simulink model "SimulationV4"  (R2018a)
settings: Solver=ode45  StartTime=0.0  StopTime=tfin  FixedStep=0.001  RelTol=1e-09  EnableMultiTasking=on
values from neighbouring files (symbols this model uses):
  A = eval(subs(A))    [CalculTFs.m]    (also in EquationCapteur.m = length(a); Modelisation.m = subs(A, [thetaeq, phieq], [0, 0]); modelisation.m = [[zeros([3,3]) eye(3) zeros([3,2]) zeros([3,2]) zeros([3,3]); run_bancessai.m)
  A_phi = [A_plaque(1,1) A_plaque(1,4) A_plaque(1,7) ... (first row only)    [CalculTFs.m]
  A_theta = [A_plaque(2,2) A_plaque(2,5) A_plaque(2,8) ... (first row only)    [CalculTFs.m]
  A_z = [A_plaque(3,3) A_plaque(3,6) A_plaque(3,9) ... (first row only)    [CalculTFs.m]
  ae0 = a2(1)    [Actionneurs.m]    (also in CoefficientsActionneurs.mat = 1.33340598826)
  ae1 = a2(2)    [Actionneurs.m]    (also in CoefficientsActionneurs.mat = 362.21410211)
  ae2 = a2(3)    [Actionneurs.m]    (also in CoefficientsActionneurs.mat = 2183.40136704)
  ae3 = a2(4)    [Actionneurs.m]    (also in CoefficientsActionneurs.mat = 705425.288236)
  as0 = a3(1)    [Actionneurs.m]    (also in CoefficientsActionneurs.mat = 0.0586667067)
  as1 = a3(2)    [Actionneurs.m]    (also in CoefficientsActionneurs.mat = 22.4105523392)
  as2 = a3(3)    [Actionneurs.m]    (also in CoefficientsActionneurs.mat = 860.394175869)
  as3 = a3(4)    [Actionneurs.m]    (also in CoefficientsActionneurs.mat = 233710.908706)
  B = eval(subs(B))    [CalculTFs.m]    (also in EquationCapteur.m = length(b); Modelisation.m = [[zeros([3,3])]; modelisation.m = [[zeros([3,3])]; run_bancessai.m)
  B_phi = [0;0;B_plaque(7,1)]    [CalculTFs.m]
  B_theta = [0;0;B_plaque(8,2)]    [CalculTFs.m]
  B_z = [0;0;B_plaque(9,3)]    [CalculTFs.m]
  be1 = 13.029359254409743    (= 13.0293592544)    [Actionneurs.m]    (also in CoefficientsActionneurs.mat)
  C = eval(subs(C))    [CalculTFs.m]    (also in EquationCapteur.m = length(c); Modelisation.m = [[Tdef zeros([3,3]) zeros([3,4]) zeros([3,3])]; modelisation.m = [[Tdef zeros([3,3]) zeros([3,4]) zeros([3,3])]; run_bancessai.m)
  C_dec = [1 0 0]    [CalculTFs.m]
  D = eval(subs(D))    [CalculTFs.m]    (also in EquationCapteur.m = length(d); Linearisation.mat = [0 0 0 0 0 0 0 0 0 0 0 0 ... (21 elements, 7x3)]; Modelisation.m = zeros([7,3]); modelisation.m = zeros([7,3]))
  D_dec = [0]    [CalculTFs.m]
  g = 9.81    [bancEssaiConstantes.m]    (also in trajectoire.m = sqrt(1 + (df).^2))
  Jx = 1169e-06    (= 0.001169)    [bancEssaiConstantes.m]
  Jy = Jx    (= 0.001169)    [bancEssaiConstantes.m]
  LA = LL    (= 0.115)    [bancEssaiConstantes.m]
  LB = LL    (= 0.115)    [bancEssaiConstantes.m]
  LC = LL    (= 0.115)    [bancEssaiConstantes.m]
  mS = 0.0080    (= 0.008)    [bancEssaiConstantes.m]
  mSeff = mS+JS/rS^2    (= 0.0112)    [bancEssaiConstantes.m]
  mtot = mP + sig*mS    [bancEssaiConstantes.m]
  Pxeq = xSeq    [equilibre.m]    (also in equilibre_cube.m)
  Pyeq = ySeq    [equilibre.m]    (also in equilibre_cube.m)
  Pzeq = .015    (= 0.015)    [run_bancessai.m]
  RA = RR    (= 3.6)    [bancEssaiConstantes.m]
  RB = RR    (= 3.6)    [bancEssaiConstantes.m]
  RC = RR    (= 3.6)    [bancEssaiConstantes.m]
  sig = 1    [run_bancessai.m]
  TDEF = [yvec_DEF'; -xvec_DEF'; ones(1,3)]    [bancEssaiConstantes.m]
  U = [YA YB YC ... (first row only)    [bancEssaiConstantes.m]
  VAeq = double(IAeq*RA)    [equilibre.m]    (also in equilibre_cube.m = double(IAeq/RA))
  VBeq = double(IBeq*RB)    [equilibre.m]    (also in equilibre_cube.m = double(IBeq/RB))
  VCeq = double(ICeq*RC)    [equilibre.m]    (also in equilibre_cube.m = double(ICeq/RC))
  Vmax = 16.0    (= 16)    [bancEssaiConstantes.m]
  XA = +rABC    (= 0.0952)    [bancEssaiConstantes.m]
  XB = -rABC*sind(30)    [bancEssaiConstantes.m]
  XC = -rABC*sind(30)    [bancEssaiConstantes.m]
  XD = +rDEF*sind(30)    [bancEssaiConstantes.m]
  XE = -rDEF    (= -0.08)    [bancEssaiConstantes.m]
  XF = +rDEF*sind(30)    [bancEssaiConstantes.m]
  YA = 0.0    (= 0)    [bancEssaiConstantes.m]
  YB = +rABC*cosd(30)    [bancEssaiConstantes.m]
  YC = -rABC*cosd(30)    [bancEssaiConstantes.m]
  YD = +rDEF*cosd(30)    [bancEssaiConstantes.m]
  YE = 0.0    (= 0)    [bancEssaiConstantes.m]
  YF = -rDEF*cosd(30)    [bancEssaiConstantes.m]
undefined symbols (not defined in the file or in its folder): A_sphere, B_sphere, C_sphere, D_sphere
(part 2 of 2)

== system SimulationV4/Asservissements2/__InputSSForSFun__ ==
  zD : Inport
  zE : Inport  Port=2
  zF : Inport  Port=3
  Axdes : Inport  Port=4
  Aydes : Inport  Port=5
  zdes : Inport  Port=6
  xdes : Inport  Port=7
  ydes : Inport  Port=8
  Px : Inport  Port=9
  Py : Inport  Port=10
  Vx : Inport  Port=11
  Vy : Inport  Port=12
  __UniqueOutportName__1__ : Outport
  __UniqueOutportName__2__ : Outport  Port=2
  __UniqueOutportName__3__ : Outport  Port=3
  __UniqueOutportName__4__ : Outport  Port=4
  __UniqueOutportName__5__ : Outport  Port=5
  __UniqueOutportName__6__ : Outport  Port=6
  __UniqueOutportName__7__ : Outport  Port=7
  __UniqueOutportName__8__ : Outport  Port=8
  __UniqueOutportName__9__ : Outport  Port=9
  __UniqueOutportName__10__ : Outport  Port=10
  __UniqueOutportName__11__ : Outport  Port=11
  __UniqueOutportName__12__ : Outport  Port=12
  wires:
  zD/1 -> __UniqueOutportName__1__/1
  zE/1 -> __UniqueOutportName__2__/1
  zF/1 -> __UniqueOutportName__3__/1
  Axdes/1 -> __UniqueOutportName__4__/1
  Aydes/1 -> __UniqueOutportName__5__/1
  zdes/1 -> __UniqueOutportName__6__/1
  xdes/1 -> __UniqueOutportName__7__/1
  ydes/1 -> __UniqueOutportName__8__/1
  Px/1 -> __UniqueOutportName__9__/1
  Py/1 -> __UniqueOutportName__10__/1
  Vx/1 -> __UniqueOutportName__11__/1
  Vy/1 -> __UniqueOutportName__12__/1

== system SimulationV4/Asservissements2/__OutputSSForSFun__ ==
  __UniqueInportName__1__ : Inport
  __UniqueInportName__2__ : Inport  Port=2
  __UniqueInportName__3__ : Inport  Port=3
  __UniqueInportName__4__ : Inport  Port=4
  __UniqueInportName__5__ : Inport  Port=5
  VAcalcule : Outport
  VBcalcule : Outport  Port=2
  VCcalcule : Outport  Port=3
  Axcalcule : Outport  Port=4
  Aycalcule : Outport  Port=5
  wires:
  __UniqueInportName__1__/1 -> VAcalcule/1
  __UniqueInportName__2__/1 -> VBcalcule/1
  __UniqueInportName__3__/1 -> VCcalcule/1
  __UniqueInportName__4__/1 -> Axcalcule/1  "Ax_des"
  __UniqueInportName__5__/1 -> Aycalcule/1  "Ay_des"

== system SimulationV4/Asservissements3/__InputSSForSFun__ ==
  zD : Inport
  zE : Inport  Port=2
  zF : Inport  Port=3
  Axdes : Inport  Port=4
  Aydes : Inport  Port=5
  zdes : Inport  Port=6
  xdes : Inport  Port=7
  ydes : Inport  Port=8
  Px : Inport  Port=9
  Py : Inport  Port=10
  Vx : Inport  Port=11
  Vy : Inport  Port=12
  __UniqueOutportName__1__ : Outport
  __UniqueOutportName__2__ : Outport  Port=2
  __UniqueOutportName__3__ : Outport  Port=3
  __UniqueOutportName__4__ : Outport  Port=4
  __UniqueOutportName__5__ : Outport  Port=5
  __UniqueOutportName__6__ : Outport  Port=6
  __UniqueOutportName__7__ : Outport  Port=7
  __UniqueOutportName__8__ : Outport  Port=8
  __UniqueOutportName__9__ : Outport  Port=9
  __UniqueOutportName__10__ : Outport  Port=10
  __UniqueOutportName__11__ : Outport  Port=11
  __UniqueOutportName__12__ : Outport  Port=12
  wires:
  zD/1 -> __UniqueOutportName__1__/1
  zE/1 -> __UniqueOutportName__2__/1
  zF/1 -> __UniqueOutportName__3__/1
  Axdes/1 -> __UniqueOutportName__4__/1
  Aydes/1 -> __UniqueOutportName__5__/1
  zdes/1 -> __UniqueOutportName__6__/1
  xdes/1 -> __UniqueOutportName__7__/1
  ydes/1 -> __UniqueOutportName__8__/1
  Px/1 -> __UniqueOutportName__9__/1
  Py/1 -> __UniqueOutportName__10__/1
  Vx/1 -> __UniqueOutportName__11__/1
  Vy/1 -> __UniqueOutportName__12__/1

== system SimulationV4/Asservissements3/__OutputSSForSFun__ ==
  __UniqueInportName__1__ : Inport
  __UniqueInportName__2__ : Inport  Port=2
  __UniqueInportName__3__ : Inport  Port=3
  __UniqueInportName__4__ : Inport  Port=4
  __UniqueInportName__5__ : Inport  Port=5
  VAcalcule : Outport
  VBcalcule : Outport  Port=2
  VCcalcule : Outport  Port=3
  Axcalcule : Outport  Port=4
  Aycalcule : Outport  Port=5
  wires:
  __UniqueInportName__1__/1 -> VAcalcule/1
  __UniqueInportName__2__/1 -> VBcalcule/1
  __UniqueInportName__3__/1 -> VCcalcule/1
  __UniqueInportName__4__/1 -> Axcalcule/1  "Ax_des"
  __UniqueInportName__5__/1 -> Aycalcule/1  "Ay_des"

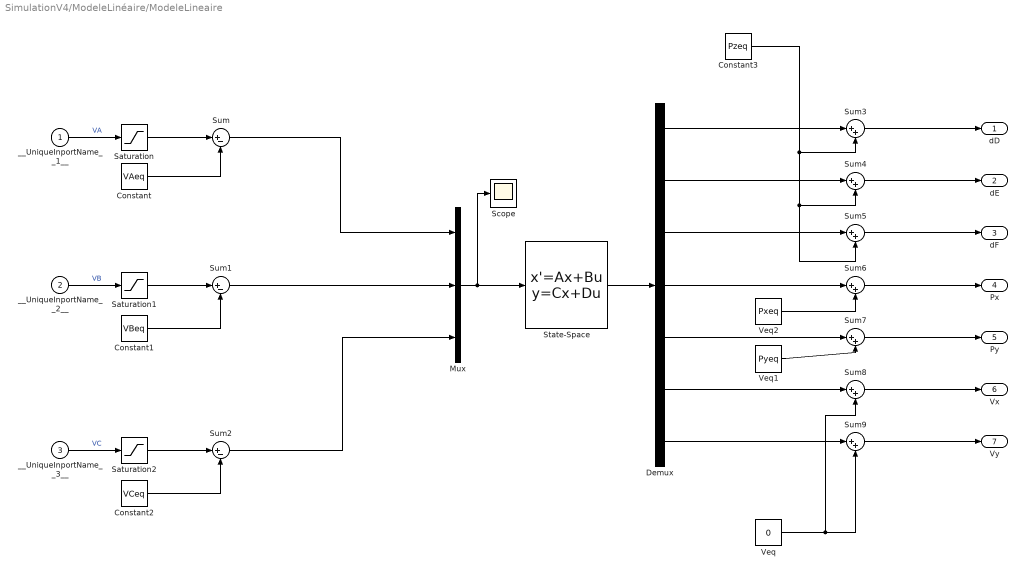
== system SimulationV4/ModeleLinéaire/ModeleLineaire ==
  __UniqueInportName__1__ : Inport
  __UniqueInportName__2__ : Inport  Port=2
  __UniqueInportName__3__ : Inport  Port=3
  Constant : Constant  Value=VAeq
  Constant1 : Constant  Value=VBeq
  Constant2 : Constant  Value=VCeq
  Constant3 : Constant  Value=Pzeq
  Demux : Demux  Outputs=7
  Mux : Mux  Inputs=3
  Saturation : Saturate  UpperLimit=Vmax  LowerLimit=-Vmax
  Saturation1 : Saturate  UpperLimit=Vmax  LowerLimit=-Vmax
  Saturation2 : Saturate  UpperLimit=Vmax  LowerLimit=-Vmax
  Scope : Scope
  State-Space : StateSpace  A=A  B=B  C=C  D=D  InitialCondition=0
  Sum : Sum  Inputs=|+-
  Sum1 : Sum  Inputs=|+-
  Sum2 : Sum  Inputs=|+-
  Sum{3..9} (7 alike) : Sum  Inputs=|++
  Veq : Constant  Value=0
  Veq1 : Constant  Value=Pyeq
  Veq2 : Constant  Value=Pxeq
  dD : Outport
  dE : Outport  Port=2
  dF : Outport  Port=3
  Px : Outport  Port=4
  Py : Outport  Port=5
  Vx : Outport  Port=6
  Vy : Outport  Port=7
  wires:
  __UniqueInportName__1__/1 -> Saturation/1  "VA"
  __UniqueInportName__2__/1 -> Saturation1/1  "VB"
  __UniqueInportName__3__/1 -> Saturation2/1  "VC"
  Mux/1 -> State-Space/1, Scope/1
  State-Space/1 -> Demux/1
  Constant/1 -> Sum/2
  Saturation/1 -> Sum/1
  Sum/1 -> Mux/1
  Saturation1/1 -> Sum1/1
  Constant1/1 -> Sum1/2
  Sum1/1 -> Mux/2
  Constant2/1 -> Sum2/2
  Sum2/1 -> Mux/3
  Saturation2/1 -> Sum2/1
  Sum3/1 -> dD/1
  Sum4/1 -> dE/1
  Sum5/1 -> dF/1
  Sum6/1 -> Px/1
  Sum7/1 -> Py/1
  Sum8/1 -> Vx/1
  Sum9/1 -> Vy/1
  Veq/1 -> Sum8/2, Sum9/2
  Demux/7 -> Sum9/1
  Demux/6 -> Sum8/1
  Veq1/1 -> Sum7/2
  Demux/5 -> Sum7/1
  Veq2/1 -> Sum6/2
  Demux/4 -> Sum6/1
  Constant3/1 -> Sum3/2, Sum4/2, Sum5/2
  Demux/1 -> Sum3/1
  Demux/2 -> Sum4/1
  Demux/3 -> Sum5/1

== system SimulationV4/ModeleLinéaire/__InputSSForSFun__ ==
  VAdesire : Inport
  VBdesire : Inport  Port=2
  VCdesire : Inport  Port=3
  __UniqueOutportName__1__ : Outport
  __UniqueOutportName__2__ : Outport  Port=2
  __UniqueOutportName__3__ : Outport  Port=3
  wires:
  VAdesire/1 -> __UniqueOutportName__1__/1
  VBdesire/1 -> __UniqueOutportName__2__/1
  VCdesire/1 -> __UniqueOutportName__3__/1

== system SimulationV4/ModeleLinéaire/__OutputSSForSFun__ ==
  __UniqueInportName__17__ : Inport
  __UniqueInportName__18__ : Inport  Port=2
  __UniqueInportName__19__ : Inport  Port=3
  __UniqueInportName__7__ : Inport  Port=4
  __UniqueInportName__8__ : Inport  Port=5
  __UniqueInportName__9__ : Inport  Port=6
  __UniqueInportName__10__ : Inport  Port=7
  zD : Outport
  zE : Outport  Port=2
  zF : Outport  Port=3
  Px : Outport  Port=4
  Py : Outport  Port=5
  Vx : Outport  Port=6
  Vy : Outport  Port=7
  wires:
  __UniqueInportName__7__/1 -> Px/1  "Px"
  __UniqueInportName__8__/1 -> Py/1  "Py"
  __UniqueInportName__9__/1 -> Vx/1  "Vx"
  __UniqueInportName__10__/1 -> Vy/1  "Vy"
  __UniqueInportName__17__/1 -> zD/1  "zd"
  __UniqueInportName__18__/1 -> zE/1  "ze"
  __UniqueInportName__19__/1 -> zF/1  "zf"

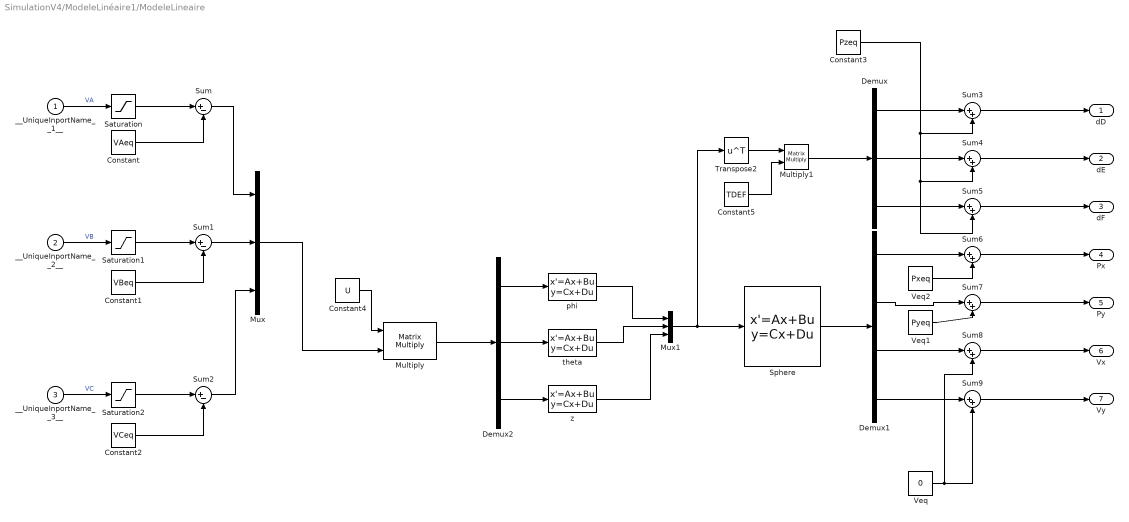
== system SimulationV4/ModeleLinéaire1/ModeleLineaire ==
  __UniqueInportName__1__ : Inport
  __UniqueInportName__2__ : Inport  Port=2
  __UniqueInportName__3__ : Inport  Port=3
  Constant : Constant  Value=VAeq
  Constant1 : Constant  Value=VBeq
  Constant2 : Constant  Value=VCeq
  Constant3 : Constant  Value=Pzeq
  Constant4 : Constant  Value=U
  Constant5 : Constant  Value=TDEF
  Demux : Demux  Outputs=3
  Demux1 : Demux
  Demux2 : Demux  Outputs=3
  Multiply : Product  Multiplication=Matrix(*)  OutDataTypeStr=Inherit: Same as first input
  Multiply1 : Product  Multiplication=Matrix(*)
  Mux : Mux  Inputs=3
  Mux1 : Mux  Inputs=3
  Saturation : Saturate  UpperLimit=Vmax  LowerLimit=-Vmax
  Saturation1 : Saturate  UpperLimit=Vmax  LowerLimit=-Vmax
  Saturation2 : Saturate  UpperLimit=Vmax  LowerLimit=-Vmax
  Sphere : StateSpace  A=A_sphere  B=B_sphere  C=C_sphere  D=D_sphere  InitialCondition=0
  Sum : Sum  Inputs=|+-
  Sum1 : Sum  Inputs=|+-
  Sum2 : Sum  Inputs=|+-
  Sum{3..9} (7 alike) : Sum  Inputs=|++
  Transpose2 : Math  Operator=transpose  SaturateOnIntegerOverflow=on
  Veq : Constant  Value=0
  Veq1 : Constant  Value=Pyeq
  Veq2 : Constant  Value=Pxeq
  phi : StateSpace  A=A_phi  B=B_phi  C=C_dec  D=D_dec  InitialCondition=0
  theta : StateSpace  A=A_theta  B=B_theta  C=C_dec  D=D_dec  InitialCondition=0
  z : StateSpace  A=A_z  B=B_z  C=C_dec  D=D_dec  InitialCondition=0
  dD : Outport
  dE : Outport  Port=2
  dF : Outport  Port=3
  Px : Outport  Port=4
  Py : Outport  Port=5
  Vx : Outport  Port=6
  Vy : Outport  Port=7
  wires:
  __UniqueInportName__1__/1 -> Saturation/1  "VA"
  __UniqueInportName__2__/1 -> Saturation1/1  "VB"
  __UniqueInportName__3__/1 -> Saturation2/1  "VC"
  Sphere/1 -> Demux1/1
  Constant/1 -> Sum/2
  Saturation/1 -> Sum/1
  Sum/1 -> Mux/1
  Saturation1/1 -> Sum1/1
  Constant1/1 -> Sum1/2
  Sum1/1 -> Mux/2
  Constant2/1 -> Sum2/2
  Sum2/1 -> Mux/3
  Saturation2/1 -> Sum2/1
  Sum3/1 -> dD/1
  Sum4/1 -> dE/1
  Sum5/1 -> dF/1
  Sum6/1 -> Px/1
  Sum7/1 -> Py/1
  Sum8/1 -> Vx/1
  Sum9/1 -> Vy/1
  Veq/1 -> Sum8/2, Sum9/2
  Demux1/4 -> Sum9/1
  Demux1/3 -> Sum8/1
  Veq1/1 -> Sum7/2
  Demux1/2 -> Sum7/1
  Veq2/1 -> Sum6/2
  Demux1/1 -> Sum6/1
  Constant3/1 -> Sum3/2, Sum4/2, Sum5/2
  Demux/1 -> Sum3/1
  Demux/2 -> Sum4/1
  Demux/3 -> Sum5/1
  Mux/1 -> Multiply/2
  Constant4/1 -> Multiply/1
  Multiply/1 -> Demux2/1
  Multiply1/1 -> Demux/1
  Constant5/1 -> Multiply1/2
  Transpose2/1 -> Multiply1/1
  Mux1/1 -> Transpose2/1, Sphere/1
  phi/1 -> Mux1/1
  theta/1 -> Mux1/2
  z/1 -> Mux1/3
  Demux2/1 -> phi/1
  Demux2/2 -> theta/1
  Demux2/3 -> z/1

== system SimulationV4/ModeleLinéaire1/__InputSSForSFun__ ==
  VAdesire : Inport
  VBdesire : Inport  Port=2
  VCdesire : Inport  Port=3
  __UniqueOutportName__1__ : Outport
  __UniqueOutportName__2__ : Outport  Port=2
  __UniqueOutportName__3__ : Outport  Port=3
  wires:
  VAdesire/1 -> __UniqueOutportName__1__/1
  VBdesire/1 -> __UniqueOutportName__2__/1
  VCdesire/1 -> __UniqueOutportName__3__/1

== system SimulationV4/ModeleLinéaire1/__OutputSSForSFun__ ==
  __UniqueInportName__17__ : Inport
  __UniqueInportName__18__ : Inport  Port=2
  __UniqueInportName__19__ : Inport  Port=3
  __UniqueInportName__7__ : Inport  Port=4
  __UniqueInportName__8__ : Inport  Port=5
  __UniqueInportName__9__ : Inport  Port=6
  __UniqueInportName__10__ : Inport  Port=7
  zD : Outport
  zE : Outport  Port=2
  zF : Outport  Port=3
  Px : Outport  Port=4
  Py : Outport  Port=5
  Vx : Outport  Port=6
  Vy : Outport  Port=7
  wires:
  __UniqueInportName__7__/1 -> Px/1  "Px"
  __UniqueInportName__8__/1 -> Py/1  "Py"
  __UniqueInportName__9__/1 -> Vx/1  "Vx"
  __UniqueInportName__10__/1 -> Vy/1  "Vy"
  __UniqueInportName__17__/1 -> zD/1  "zd"
  __UniqueInportName__18__/1 -> zE/1  "ze"
  __UniqueInportName__19__/1 -> zF/1  "zf"

== system SimulationV4/ModeleNonLineaire/__InputSSForSFun__ ==
  VAdesire : Inport
  VBdesire : Inport  Port=2
  VCdesire : Inport  Port=3
  __UniqueOutportName__1__ : Outport
  __UniqueOutportName__2__ : Outport  Port=2
  __UniqueOutportName__3__ : Outport  Port=3
  wires:
  VAdesire/1 -> __UniqueOutportName__1__/1
  VBdesire/1 -> __UniqueOutportName__2__/1
  VCdesire/1 -> __UniqueOutportName__3__/1

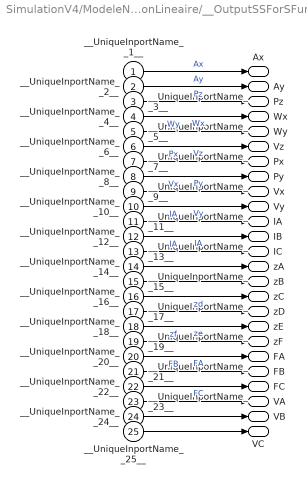
== system SimulationV4/ModeleNonLineaire/__OutputSSForSFun__ ==
  __UniqueInportName__1__ : Inport
  __UniqueInportName__2__ : Inport  Port=2
  __UniqueInportName__3__ : Inport  Port=3
  __UniqueInportName__4__ : Inport  Port=4
  __UniqueInportName__5__ : Inport  Port=5
  __UniqueInportName__6__ : Inport  Port=6
  __UniqueInportName__7__ : Inport  Port=7
  __UniqueInportName__8__ : Inport  Port=8
  __UniqueInportName__9__ : Inport  Port=9
  __UniqueInportName__10__ : Inport  Port=10
  __UniqueInportName__11__ : Inport  Port=11
  __UniqueInportName__12__ : Inport  Port=12
  __UniqueInportName__13__ : Inport  Port=13
  __UniqueInportName__14__ : Inport  Port=14
  __UniqueInportName__15__ : Inport  Port=15
  __UniqueInportName__16__ : Inport  Port=16
  __UniqueInportName__17__ : Inport  Port=17
  __UniqueInportName__18__ : Inport  Port=18
  __UniqueInportName__19__ : Inport  Port=19
  __UniqueInportName__20__ : Inport  Port=20
  __UniqueInportName__21__ : Inport  Port=21
  __UniqueInportName__22__ : Inport  Port=22
  __UniqueInportName__23__ : Inport  Port=23
  __UniqueInportName__24__ : Inport  Port=24
  __UniqueInportName__25__ : Inport  Port=25
  Ax : Outport
  Ay : Outport  Port=2
  Pz : Outport  Port=3
  Wx : Outport  Port=4
  Wy : Outport  Port=5
  Vz : Outport  Port=6
  Px : Outport  Port=7
  Py : Outport  Port=8
  Vx : Outport  Port=9
  Vy : Outport  Port=10
  IA : Outport  Port=11
  IB : Outport  Port=12
  IC : Outport  Port=13
  zA : Outport  Port=14
  zB : Outport  Port=15
  zC : Outport  Port=16
  zD : Outport  Port=17
  zE : Outport  Port=18
  zF : Outport  Port=19
  FA : Outport  Port=20
  FB : Outport  Port=21
  FC : Outport  Port=22
  VA : Outport  Port=23
  VB : Outport  Port=24
  VC : Outport  Port=25
  wires:
  __UniqueInportName__1__/1 -> Ax/1  "Ax"
  __UniqueInportName__2__/1 -> Ay/1  "Ay"
  __UniqueInportName__3__/1 -> Pz/1  "Pz"
  __UniqueInportName__4__/1 -> Wx/1  "Wx"
  __UniqueInportName__5__/1 -> Wy/1  "Wy"
  __UniqueInportName__6__/1 -> Vz/1  "Vz"
  __UniqueInportName__7__/1 -> Px/1  "Px"
  __UniqueInportName__8__/1 -> Py/1  "Py"
  __UniqueInportName__9__/1 -> Vx/1  "Vx"
  __UniqueInportName__10__/1 -> Vy/1  "Vy"
  __UniqueInportName__11__/1 -> IA/1  "IA"
  __UniqueInportName__12__/1 -> IB/1  "IA"
  __UniqueInportName__13__/1 -> IC/1  "IA"
  __UniqueInportName__14__/1 -> zA/1
  __UniqueInportName__15__/1 -> zB/1
  __UniqueInportName__16__/1 -> zC/1
  __UniqueInportName__17__/1 -> zD/1  "zd"
  __UniqueInportName__18__/1 -> zE/1  "ze"
  __UniqueInportName__19__/1 -> zF/1  "zf"
  __UniqueInportName__20__/1 -> FA/1  "FA"
  __UniqueInportName__21__/1 -> FB/1  "FB"
  __UniqueInportName__22__/1 -> FC/1  "FC"
  __UniqueInportName__23__/1 -> VA/1
  __UniqueInportName__24__/1 -> VB/1
  __UniqueInportName__25__/1 -> VC/1

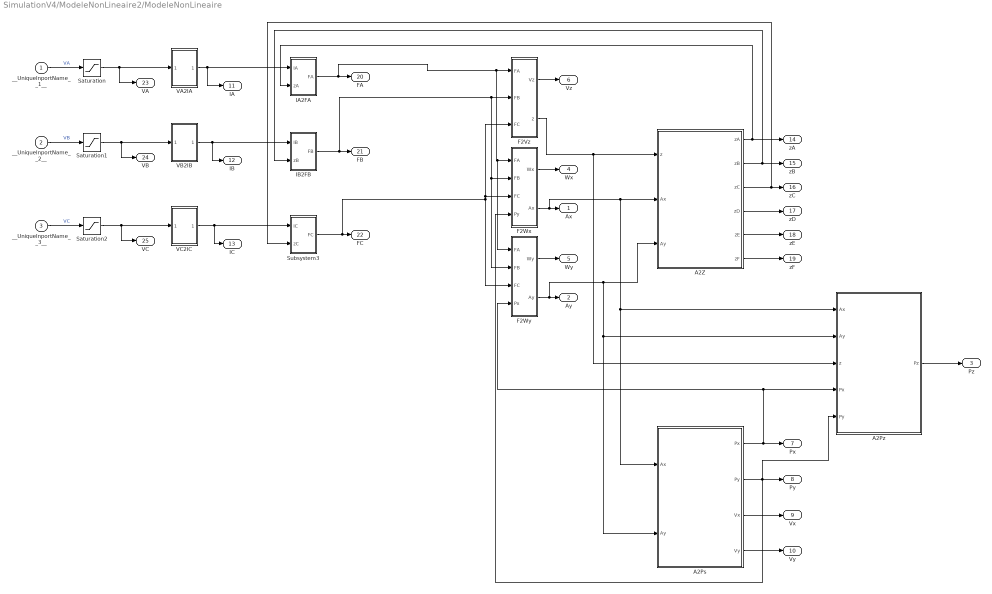
== system SimulationV4/ModeleNonLineaire2/ModeleNonLineaire ==
  __UniqueInportName__1__ : Inport
  __UniqueInportName__2__ : Inport  Port=2
  __UniqueInportName__3__ : Inport  Port=3
  A2Ps : Subsystem
  A2Pz : Subsystem
  A2Z : Subsystem
  F2Vz : Subsystem
  F2Wx : Subsystem
  F2Wy : Subsystem
  IA2FA : Subsystem
  IB2FB : Subsystem
  Saturation : Saturate  UpperLimit=Vmax  LowerLimit=-Vmax
  Saturation1 : Saturate  UpperLimit=Vmax  LowerLimit=-Vmax
  Saturation2 : Saturate  UpperLimit=Vmax  LowerLimit=-Vmax
  Subsystem3 : Subsystem
  VA2IA : Subsystem
  VB2IB : Subsystem
  VC2IC : Subsystem
  Ax : Outport
  Ay : Outport  Port=2
  Pz : Outport  Port=3
  Wx : Outport  Port=4
  Wy : Outport  Port=5
  Vz : Outport  Port=6
  Px : Outport  Port=7
  Py : Outport  Port=8
  Vx : Outport  Port=9
  Vy : Outport  Port=10
  IA : Outport  Port=11
  IB : Outport  Port=12
  IC : Outport  Port=13
  zA : Outport  Port=14
  zB : Outport  Port=15
  zC : Outport  Port=16
  zD : Outport  Port=17
  zE : Outport  Port=18
  zF : Outport  Port=19
  FA : Outport  Port=20
  FB : Outport  Port=21
  FC : Outport  Port=22
  VA : Outport  Port=23
  VB : Outport  Port=24
  VC : Outport  Port=25
  wires:
  __UniqueInportName__1__/1 -> Saturation/1  "VA"
  __UniqueInportName__2__/1 -> Saturation1/1  "VB"
  __UniqueInportName__3__/1 -> Saturation2/1  "VC"
  Saturation/1 -> VA2IA/1(In1), VA/1
  VA2IA/1(Out1) -> IA2FA/1(IA), IA/1
  Saturation1/1 -> VB2IB/1(In1), VB/1
  VB2IB/1(Out1) -> IB/1, IB2FB/1(IB)
  Saturation2/1 -> VC2IC/1(In1), VC/1
  VC2IC/1(Out1) -> Subsystem3/1(IC), IC/1
  F2Vz/1(Vz) -> Vz/1
  F2Wx/1(Wx) -> Wx/1
  F2Wy/1(Wy) -> Wy/1
  IA2FA/1(FA) -> F2Wy/1(FA), F2Wx/1(FA), F2Vz/1(FA), FA/1
  Subsystem3/1(FC) -> F2Vz/3(FC), F2Wx/3(FC), F2Wy/3(FC), FC/1
  IB2FB/1(FB) -> F2Wy/2(FB), F2Wx/2(FB), F2Vz/2(FB), FB/1
  F2Wy/2(Ay) -> A2Ps/2(Ay), A2Pz/2(Ay), A2Z/3(Ay), Ay/1
  F2Vz/2(z) -> A2Pz/3(z), A2Z/1(z)
  F2Wx/2(Ax) -> A2Pz/1(Ax), A2Ps/1(Ax), A2Z/2(Ax), Ax/1
  A2Z/1(zA) -> zA/1, IA2FA/2(zA)
  A2Z/2(zB) -> IB2FB/2(zB), zB/1
  A2Z/3(zC) -> Subsystem3/2(zC), zC/1
  A2Z/4(zD) -> zD/1
  A2Z/5(zE) -> zE/1
  A2Z/6(zF) -> zF/1
  A2Ps/2(Py) -> A2Pz/5(Py), F2Wx/4(Py), Py/1
  A2Ps/3(Vx) -> Vx/1
  A2Ps/4(Vy) -> Vy/1
  A2Pz/1(Pz) -> Pz/1
  A2Ps/1(Px) -> A2Pz/4(Px), F2Wy/4(Px), Px/1

== system SimulationV4/ModeleNonLineaire2/__InputSSForSFun__ ==
  VAdesire : Inport
  VBdesire : Inport  Port=2
  VCdesire : Inport  Port=3
  __UniqueOutportName__1__ : Outport
  __UniqueOutportName__2__ : Outport  Port=2
  __UniqueOutportName__3__ : Outport  Port=3
  wires:
  VAdesire/1 -> __UniqueOutportName__1__/1
  VBdesire/1 -> __UniqueOutportName__2__/1
  VCdesire/1 -> __UniqueOutportName__3__/1

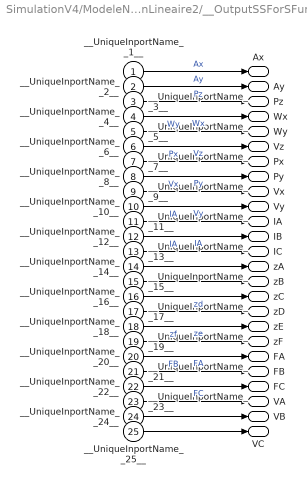
== system SimulationV4/ModeleNonLineaire2/__OutputSSForSFun__ ==
  __UniqueInportName__1__ : Inport
  __UniqueInportName__2__ : Inport  Port=2
  __UniqueInportName__3__ : Inport  Port=3
  __UniqueInportName__4__ : Inport  Port=4
  __UniqueInportName__5__ : Inport  Port=5
  __UniqueInportName__6__ : Inport  Port=6
  __UniqueInportName__7__ : Inport  Port=7
  __UniqueInportName__8__ : Inport  Port=8
  __UniqueInportName__9__ : Inport  Port=9
  __UniqueInportName__10__ : Inport  Port=10
  __UniqueInportName__11__ : Inport  Port=11
  __UniqueInportName__12__ : Inport  Port=12
  __UniqueInportName__13__ : Inport  Port=13
  __UniqueInportName__14__ : Inport  Port=14
  __UniqueInportName__15__ : Inport  Port=15
  __UniqueInportName__16__ : Inport  Port=16
  __UniqueInportName__17__ : Inport  Port=17
  __UniqueInportName__18__ : Inport  Port=18
  __UniqueInportName__19__ : Inport  Port=19
  __UniqueInportName__20__ : Inport  Port=20
  __UniqueInportName__21__ : Inport  Port=21
  __UniqueInportName__22__ : Inport  Port=22
  __UniqueInportName__23__ : Inport  Port=23
  __UniqueInportName__24__ : Inport  Port=24
  __UniqueInportName__25__ : Inport  Port=25
  Ax : Outport
  Ay : Outport  Port=2
  Pz : Outport  Port=3
  Wx : Outport  Port=4
  Wy : Outport  Port=5
  Vz : Outport  Port=6
  Px : Outport  Port=7
  Py : Outport  Port=8
  Vx : Outport  Port=9
  Vy : Outport  Port=10
  IA : Outport  Port=11
  IB : Outport  Port=12
  IC : Outport  Port=13
  zA : Outport  Port=14
  zB : Outport  Port=15
  zC : Outport  Port=16
  zD : Outport  Port=17
  zE : Outport  Port=18
  zF : Outport  Port=19
  FA : Outport  Port=20
  FB : Outport  Port=21
  FC : Outport  Port=22
  VA : Outport  Port=23
  VB : Outport  Port=24
  VC : Outport  Port=25
  wires:
  __UniqueInportName__1__/1 -> Ax/1  "Ax"
  __UniqueInportName__2__/1 -> Ay/1  "Ay"
  __UniqueInportName__3__/1 -> Pz/1  "Pz"
  __UniqueInportName__4__/1 -> Wx/1  "Wx"
  __UniqueInportName__5__/1 -> Wy/1  "Wy"
  __UniqueInportName__6__/1 -> Vz/1  "Vz"
  __UniqueInportName__7__/1 -> Px/1  "Px"
  __UniqueInportName__8__/1 -> Py/1  "Py"
  __UniqueInportName__9__/1 -> Vx/1  "Vx"
  __UniqueInportName__10__/1 -> Vy/1  "Vy"
  __UniqueInportName__11__/1 -> IA/1  "IA"
  __UniqueInportName__12__/1 -> IB/1  "IA"
  __UniqueInportName__13__/1 -> IC/1  "IA"
  __UniqueInportName__14__/1 -> zA/1
  __UniqueInportName__15__/1 -> zB/1
  __UniqueInportName__16__/1 -> zC/1
  __UniqueInportName__17__/1 -> zD/1  "zd"
  __UniqueInportName__18__/1 -> zE/1  "ze"
  __UniqueInportName__19__/1 -> zF/1  "zf"
  __UniqueInportName__20__/1 -> FA/1  "FA"
  __UniqueInportName__21__/1 -> FB/1  "FB"
  __UniqueInportName__22__/1 -> FC/1  "FC"
  __UniqueInportName__23__/1 -> VA/1
  __UniqueInportName__24__/1 -> VB/1
  __UniqueInportName__25__/1 -> VC/1

== system SimulationV4/Asservissements1/Subsystem/Ax ==
  zd : Inport
  zf : Inport  Port=2
  Constant : Constant  Value=25*sqrt(3)/6
  Multiply : Product
  Subtract : Sum  Inputs=+-
  Ax : Outport
  wires:
  zd/1 -> Subtract/1
  zf/1 -> Subtract/2
  Subtract/1 -> Multiply/1
  Constant/1 -> Multiply/2
  Multiply/1 -> Ax/1

== system SimulationV4/Asservissements1/Subsystem/Ay ==
  zd : Inport
  ze : Inport  Port=2
  zf : Inport  Port=3
  Constant : Constant  Value=2
  Constant1 : Constant  Value=25/3
  Divide : Product  Inputs=*/
  Multiply : Product
  Subtract : Sum  Inputs=+-
  Sum : Sum  Inputs=|++
  Ay : Outport
  wires:
  zf/1 -> Sum/2
  zd/1 -> Sum/1
  Sum/1 -> Divide/1
  Constant/1 -> Divide/2
  Subtract/1 -> Multiply/1
  Constant1/1 -> Multiply/2
  Multiply/1 -> Ay/1
  ze/1 -> Subtract/1
  Divide/1 -> Subtract/2

== system SimulationV4/Asservissements1/Subsystem/z0 ==
  zd : Inport
  ze : Inport  Port=2
  zf : Inport  Port=3
  Constant : Constant  Value=3
  Divide : Product  Inputs=*/
  Sum : Sum  Inputs=3
  z0 : Outport
  wires:
  ze/1 -> Sum/2
  zd/1 -> Sum/1
  Sum/1 -> Divide/1
  zf/1 -> Sum/3
  Constant/1 -> Divide/2
  Divide/1 -> z0/1

== system SimulationV4/ModeleNonLineaire2/ModeleNonLineaire/A2Ps ==
  Ax : Inport
  Ay : Inport  Port=2
  Gain : Gain  Gain=mS*sig*g/mSeff
  Gain1 : Gain  Gain=-mS*sig*g/mSeff
  Integrator{,1..3} (4 alike) : Integrator
  Px : Outport
  Py : Outport  Port=2
  Vx : Outport  Port=3
  Vy : Outport  Port=4
  wires:
  Ax/1 -> Gain/1
  Ay/1 -> Gain1/1
  Gain/1 -> Integrator/1
  Gain1/1 -> Integrator1/1
  Integrator1/1 -> Vx/1, Integrator3/1
  Integrator/1 -> Vy/1, Integrator2/1
  Integrator2/1 -> Py/1
  Integrator3/1 -> Px/1

== system SimulationV4/ModeleNonLineaire2/ModeleNonLineaire/A2Pz ==
  Ax : Inport
  Ay : Inport  Port=2
  z : Inport  Port=3
  Px : Inport  Port=4
  Py : Inport  Port=5
  Add : Sum  Inputs=+-+
  Product : Product
  Product1 : Product
  Pz : Outport
  wires:
  Ax/1 -> Product/1
  Ay/1 -> Product1/1
  Px/1 -> Product1/2
  Py/1 -> Product/2
  z/1 -> Add/3
  Add/1 -> Pz/1

== system SimulationV4/ModeleNonLineaire2/ModeleNonLineaire/A2Z ==
  z : Inport
  Ax : Inport  Port=2
  Ay : Inport  Port=3
  Gain : Gain  Gain=YA
  Gain1 : Gain  Gain=XA
  Gain10 : Gain  Gain=YF
  Gain11 : Gain  Gain=XF
  Gain2 : Gain  Gain=YB
  Gain3 : Gain  Gain=XB
  Gain4 : Gain  Gain=YC
  Gain5 : Gain  Gain=XC
  Gain6 : Gain  Gain=YD
  Gain7 : Gain  Gain=XD
  Gain8 : Gain  Gain=YE
  Gain9 : Gain  Gain=XE
  Subtract{,1..5} (6 alike) : Sum  Inputs=++-
  zA : Outport
  zB : Outport  Port=2
  zC : Outport  Port=3
  zD : Outport  Port=4
  zE : Outport  Port=5
  zF : Outport  Port=6
  wires:
  Gain/1 -> Subtract/2
  Gain1/1 -> Subtract/3
  Subtract/1 -> zA/1
  Gain2/1 -> Subtract1/2
  Gain3/1 -> Subtract1/3
  Subtract1/1 -> zB/1
  Gain4/1 -> Subtract2/2
  Gain5/1 -> Subtract2/3
  Subtract2/1 -> zC/1
  Gain6/1 -> Subtract3/2
  Gain7/1 -> Subtract3/3
  Subtract3/1 -> zD/1
  Gain8/1 -> Subtract4/2
  Gain9/1 -> Subtract4/3
  Subtract4/1 -> zE/1
  Gain10/1 -> Subtract5/2
  Gain11/1 -> Subtract5/3
  Subtract5/1 -> zF/1
  z/1 -> Subtract5/1, Subtract4/1, Subtract3/1, Subtract2/1, Subtract1/1, Subtract/1
  Ax/1 -> Gain10/1, Gain8/1, Gain6/1, Gain4/1, Gain2/1, Gain/1
  Ay/1 -> Gain11/1, Gain9/1, Gain7/1, Gain5/1, Gain3/1, Gain1/1

== system SimulationV4/ModeleNonLineaire2/ModeleNonLineaire/F2Vz ==
  FA : Inport
  FB : Inport  Port=2
  FC : Inport  Port=3
  Add : Sum  Inputs=++++
  Constant : Constant  Value=g
  Gain : Gain  Gain=1/mtot
  Gain1 : Gain  Gain=1/mtot
  Gain2 : Gain  Gain=1/mtot
  Integrator : Integrator
  Integrator1 : Integrator  InitialCondition=Pzeq
  Vz : Outport
  z : Outport  Port=2
  wires:
  Constant/1 -> Add/1
  FA/1 -> Gain/1
  FB/1 -> Gain1/1
  FC/1 -> Gain2/1
  Gain2/1 -> Add/4
  Gain1/1 -> Add/3
  Gain/1 -> Add/2
  Add/1 -> Integrator/1
  Integrator/1 -> Integrator1/1, Vz/1
  Integrator1/1 -> z/1

== system SimulationV4/ModeleNonLineaire2/ModeleNonLineaire/F2Wx ==
  FA : Inport
  FB : Inport  Port=2
  FC : Inport  Port=3
  Py : Inport  Port=4
  Add : Sum  Inputs=++++
  Gain : Gain  Gain=YA/Jx
  Gain1 : Gain  Gain=YB/Jx
  Gain2 : Gain  Gain=YC/Jx
  Gain3 : Gain  Gain=mS*sig*g/Jx
  Integrator : Integrator
  Integrator1 : Integrator
  Wx : Outport
  Ax : Outport  Port=2
  wires:
  FA/1 -> Gain/1
  FB/1 -> Gain1/1
  FC/1 -> Gain2/1
  Add/1 -> Integrator/1
  Integrator/1 -> Integrator1/1, Wx/1
  Py/1 -> Gain3/1
  Gain3/1 -> Add/4
  Gain2/1 -> Add/3
  Gain1/1 -> Add/2
  Gain/1 -> Add/1
  Integrator1/1 -> Ax/1

== system SimulationV4/ModeleNonLineaire2/ModeleNonLineaire/F2Wy ==
  FA : Inport
  FB : Inport  Port=2
  FC : Inport  Port=3
  Px : Inport  Port=4
  Add : Sum  Inputs=++++
  Gain : Gain  Gain=-XA/Jy
  Gain1 : Gain  Gain=-XB/Jy
  Gain2 : Gain  Gain=-XC/Jy
  Gain3 : Gain  Gain=-mS*sig*g/Jy
  Integrator : Integrator
  Integrator1 : Integrator
  Wy : Outport
  Ay : Outport  Port=2
  wires:
  FA/1 -> Gain/1
  FB/1 -> Gain1/1
  FC/1 -> Gain2/1
  Add/1 -> Integrator/1
  Integrator/1 -> Integrator1/1, Wy/1
  Px/1 -> Gain3/1
  Gain3/1 -> Add/4
  Gain2/1 -> Add/3
  Gain1/1 -> Add/2
  Gain/1 -> Add/1
  Integrator1/1 -> Ay/1

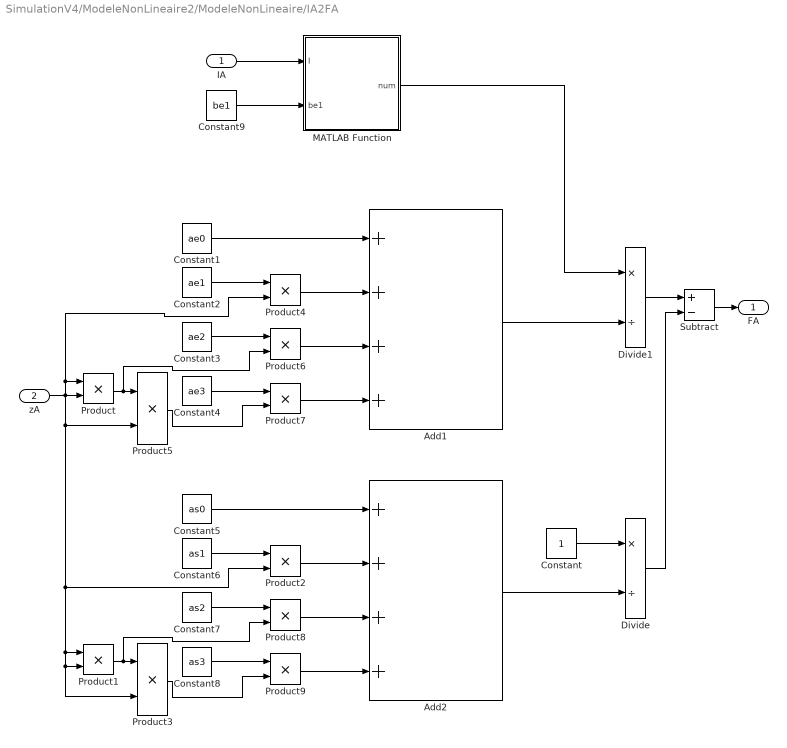
== system SimulationV4/ModeleNonLineaire2/ModeleNonLineaire/IA2FA ==
  IA : Inport
  zA : Inport  Port=2
  Add1 : Sum  Inputs=++++
  Add2 : Sum  Inputs=++++
  Constant : Constant
  Constant1 : Constant  Value=ae0
  Constant2 : Constant  Value=ae1
  Constant3 : Constant  Value=ae2
  Constant4 : Constant  Value=ae3
  Constant5 : Constant  Value=as0
  Constant6 : Constant  Value=as1
  Constant7 : Constant  Value=as2
  Constant8 : Constant  Value=as3
  Constant9 : Constant  Value=be1
  Divide : Product  Inputs=*/
  Divide1 : Product  Inputs=*/
  MATLAB Function : MATLAB Function  TreatAsAtomicUnit=on
  Product{,1..9} (10 alike) : Product
  Subtract : Sum  Inputs=+-
  FA : Outport
  wires:
  Product/1 -> Product6/2, Product5/1
  Constant1/1 -> Add1/1
  Constant2/1 -> Product4/1
  Product4/1 -> Add1/2
  Constant3/1 -> Product6/1
  Product6/1 -> Add1/3
  Constant4/1 -> Product7/1
  Product5/1 -> Product7/2
  Product7/1 -> Add1/4
  Product1/1 -> Product8/2, Product3/1
  Constant5/1 -> Add2/1
  Constant6/1 -> Product2/1
  Product2/1 -> Add2/2
  Constant7/1 -> Product8/1
  Product8/1 -> Add2/3
  Constant8/1 -> Product9/1
  Product3/1 -> Product9/2
  Product9/1 -> Add2/4
  zA/1 -> Product4/2, Product/1, Product3/2, Product1/2, Product1/1, Product2/2, Product5/2, Product/2
  Constant/1 -> Divide/1
  Add2/1 -> Divide/2
  Add1/1 -> Divide1/2
  Divide1/1 -> Subtract/1
  Subtract/1 -> FA/1
  Divide/1 -> Subtract/2
  Constant9/1 -> MATLAB Function/2(be1)
  IA/1 -> MATLAB Function/1(I)
  MATLAB Function/1(num) -> Divide1/1

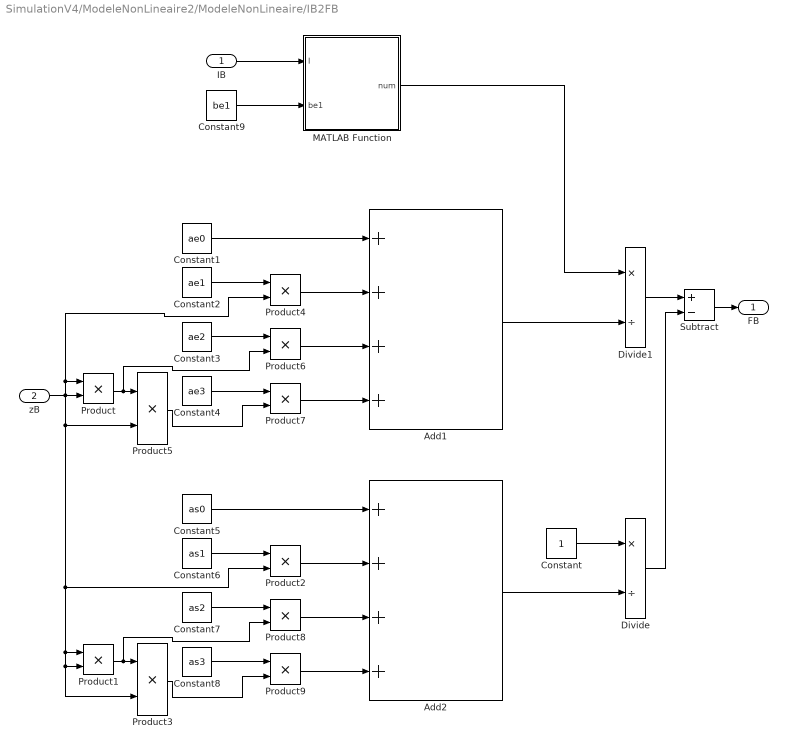
== system SimulationV4/ModeleNonLineaire2/ModeleNonLineaire/IB2FB ==
  IB : Inport
  zB : Inport  Port=2
  Add1 : Sum  Inputs=++++
  Add2 : Sum  Inputs=++++
  Constant : Constant
  Constant1 : Constant  Value=ae0
  Constant2 : Constant  Value=ae1
  Constant3 : Constant  Value=ae2
  Constant4 : Constant  Value=ae3
  Constant5 : Constant  Value=as0
  Constant6 : Constant  Value=as1
  Constant7 : Constant  Value=as2
  Constant8 : Constant  Value=as3
  Constant9 : Constant  Value=be1
  Divide : Product  Inputs=*/
  Divide1 : Product  Inputs=*/
  MATLAB Function : MATLAB Function  TreatAsAtomicUnit=on
  Product{,1..9} (10 alike) : Product
  Subtract : Sum  Inputs=+-
  FB : Outport
  wires:
  Product/1 -> Product6/2, Product5/1
  Constant1/1 -> Add1/1
  Constant2/1 -> Product4/1
  Product4/1 -> Add1/2
  Constant3/1 -> Product6/1
  Product6/1 -> Add1/3
  Constant4/1 -> Product7/1
  Product5/1 -> Product7/2
  Product7/1 -> Add1/4
  Product1/1 -> Product8/2, Product3/1
  Constant5/1 -> Add2/1
  Constant6/1 -> Product2/1
  Product2/1 -> Add2/2
  Constant7/1 -> Product8/1
  Product8/1 -> Add2/3
  Constant8/1 -> Product9/1
  Product3/1 -> Product9/2
  Product9/1 -> Add2/4
  zB/1 -> Product4/2, Product/1, Product3/2, Product1/2, Product1/1, Product2/2, Product5/2, Product/2
  Constant/1 -> Divide/1
  Add2/1 -> Divide/2
  Add1/1 -> Divide1/2
  Divide1/1 -> Subtract/1
  Subtract/1 -> FB/1
  Divide/1 -> Subtract/2
  Constant9/1 -> MATLAB Function/2(be1)
  IB/1 -> MATLAB Function/1(I)
  MATLAB Function/1(num) -> Divide1/1

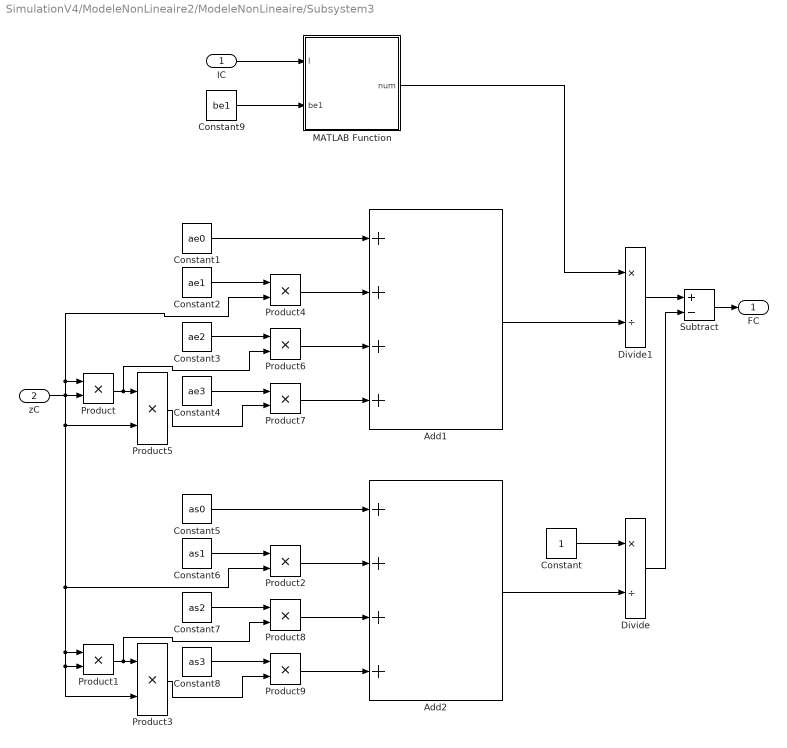
== system SimulationV4/ModeleNonLineaire2/ModeleNonLineaire/Subsystem3 ==
  IC : Inport
  zC : Inport  Port=2
  Add1 : Sum  Inputs=++++
  Add2 : Sum  Inputs=++++
  Constant : Constant
  Constant1 : Constant  Value=ae0
  Constant2 : Constant  Value=ae1
  Constant3 : Constant  Value=ae2
  Constant4 : Constant  Value=ae3
  Constant5 : Constant  Value=as0
  Constant6 : Constant  Value=as1
  Constant7 : Constant  Value=as2
  Constant8 : Constant  Value=as3
  Constant9 : Constant  Value=be1
  Divide : Product  Inputs=*/
  Divide1 : Product  Inputs=*/
  MATLAB Function : MATLAB Function  TreatAsAtomicUnit=on
  Product{,1..9} (10 alike) : Product
  Subtract : Sum  Inputs=+-
  FC : Outport
  wires:
  Product/1 -> Product6/2, Product5/1
  Constant1/1 -> Add1/1
  Constant2/1 -> Product4/1
  Product4/1 -> Add1/2
  Constant3/1 -> Product6/1
  Product6/1 -> Add1/3
  Constant4/1 -> Product7/1
  Product5/1 -> Product7/2
  Product7/1 -> Add1/4
  Product1/1 -> Product8/2, Product3/1
  Constant5/1 -> Add2/1
  Constant6/1 -> Product2/1
  Product2/1 -> Add2/2
  Constant7/1 -> Product8/1
  Product8/1 -> Add2/3
  Constant8/1 -> Product9/1
  Product3/1 -> Product9/2
  Product9/1 -> Add2/4
  zC/1 -> Product4/2, Product/1, Product3/2, Product1/2, Product1/1, Product2/2, Product5/2, Product/2
  Constant/1 -> Divide/1
  Add2/1 -> Divide/2
  Add1/1 -> Divide1/2
  Divide1/1 -> Subtract/1
  Subtract/1 -> FC/1
  Divide/1 -> Subtract/2
  Constant9/1 -> MATLAB Function/2(be1)
  IC/1 -> MATLAB Function/1(I)
  MATLAB Function/1(num) -> Divide1/1

== system SimulationV4/ModeleNonLineaire2/ModeleNonLineaire/VA2IA ==
  In1 : Inport
  Gain : Gain  Gain=1/LA
  Gain1 : Gain  Gain=RA/LA
  Integrator : Integrator  InitialCondition=-0.496058088227384
  Subtract : Sum  Inputs=+-
  Out1 : Outport
  wires:
  In1/1 -> Gain/1
  Integrator/1 -> Out1/1, Gain1/1
  Subtract/1 -> Integrator/1
  Gain/1 -> Subtract/1
  Gain1/1 -> Subtract/2

== system SimulationV4/ModeleNonLineaire2/ModeleNonLineaire/VB2IB ==
  In1 : Inport
  Gain : Gain  Gain=1/LB
  Gain1 : Gain  Gain=RB/LB
  Integrator : Integrator  InitialCondition=-0.496058088227384
  Subtract : Sum  Inputs=+-
  Out1 : Outport
  wires:
  In1/1 -> Gain/1
  Integrator/1 -> Out1/1, Gain1/1
  Subtract/1 -> Integrator/1
  Gain/1 -> Subtract/1
  Gain1/1 -> Subtract/2

== system SimulationV4/ModeleNonLineaire2/ModeleNonLineaire/VC2IC ==
  In1 : Inport
  Gain : Gain  Gain=1/LC
  Gain1 : Gain  Gain=RC/LC
  Integrator : Integrator  InitialCondition=-0.496058088227384
  Subtract : Sum  Inputs=+-
  Out1 : Outport
  wires:
  In1/1 -> Gain/1
  Integrator/1 -> Out1/1, Gain1/1
  Subtract/1 -> Integrator/1
  Gain/1 -> Subtract/1
  Gain1/1 -> Subtract/2

== matlab function SimulationV4/ModeleNonLineaire2/ModeleNonLineaire/IA2FA/MATLAB Function ==
  data: I input; num output; be1 input
function num = fcn(I,be1)
%#codegen

num = (I^2+be1*abs(I))*sign(I);

== matlab function SimulationV4/ModeleNonLineaire2/ModeleNonLineaire/IB2FB/MATLAB Function ==
  data: I input; num output; be1 input
function num = fcn(I,be1)
%#codegen

num = (I^2+be1*abs(I))*sign(I);

== matlab function SimulationV4/ModeleNonLineaire2/ModeleNonLineaire/Subsystem3/MATLAB Function ==
  data: I input; num output; be1 input
function num = fcn(I,be1)
%#codegen

num = (I^2+be1*abs(I))*sign(I);
